simulink model "questD_Luenberger_model"  (R2018a)
settings: Solver=VariableStepAuto  StartTime=0.0  StopTime=14  RelTol=1e-3
values from neighbouring files (symbols this model uses):
  A = [0 1 0 0; 20.6 0 0 0; 0 0 0 1; -.5 0 0 0]    [InvertedPendulum.m]
  B = [0; -1; 0; .5]    [InvertedPendulum.m]
  C = [1 0 0 0; 0 0 1 0]    [InvertedPendulum.m]
  K = place(A, B, p)    [InvertedPendulum.m]
  L = place(A', C', obv_poles)'    [InvertedPendulum.m]
  x0 = [-.2; -.06; .01; .3]    [InvertedPendulum.m]
settings Model: Creator=patsa  LastModifiedBy=patsa

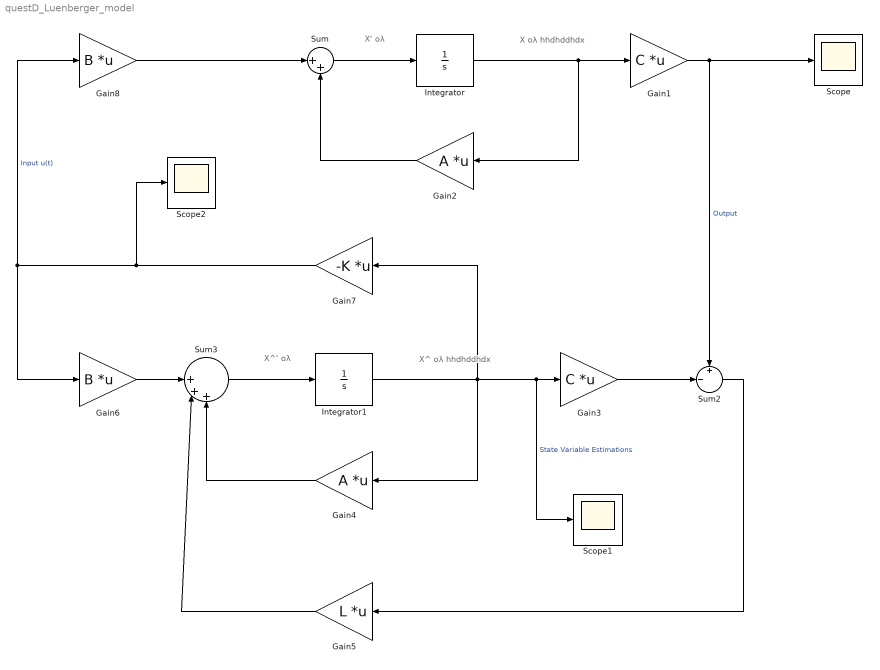
== system questD_Luenberger_model ==
  note: X' ολ
  note: X ολ
      |
      | hhdhddhdx
  note: X^' ολ
  note: X^ ολ
      |
      | hhdhddhdx
  Gain1 : Gain  Gain=C  Multiplication=Matrix(K*u)
  Gain2 : Gain  Gain=A  Multiplication=Matrix(K*u)
  Gain3 : Gain  Gain=C  Multiplication=Matrix(K*u)
  Gain4 : Gain  Gain=A  Multiplication=Matrix(K*u)
  Gain5 : Gain  Gain=L  Multiplication=Matrix(K*u)
  Gain6 : Gain  Gain=B  Multiplication=Matrix(K*u)
  Gain7 : Gain  Gain=-K  Multiplication=Matrix(K*u)
  Gain8 : Gain  Gain=B  Multiplication=Matrix(K*u)
  Integrator : Integrator  InitialCondition=x0
  Integrator1 : Integrator
  Scope : Scope
  Scope1 : Scope
  Scope2 : Scope
  Sum : Sum  Inputs=|++
  Sum2 : Sum  Inputs=+|-||
  Sum3 : Sum  Inputs=||||+|+|+
  wires:
  Gain1/1 -> Sum2/1, Scope/1  "Output"
  Gain2/1 -> Sum/2
  Integrator/1 -> Gain1/1, Gain2/1
  Sum/1 -> Integrator/1
  Integrator1/1 -> Gain7/1, Scope1/1, Gain3/1, Gain4/1  "State Variable Estimations"
  Gain3/1 -> Sum2/2
  Sum2/1 -> Gain5/1
  Gain6/1 -> Sum3/1
  Sum3/1 -> Integrator1/1
  Gain4/1 -> Sum3/3
  Gain5/1 -> Sum3/2
  Gain8/1 -> Sum/1
  Gain7/1 -> Scope2/1, Gain8/1, Gain6/1  "Input u(t)"
